simulink model "vectorTest"  (R2020a)
settings: Solver=FixedStepDiscrete  StartTime=0.0  StopTime=10.0  RelTol=1e-3
settings Model: Creator=cyarp  LastModifiedBy=cyarp

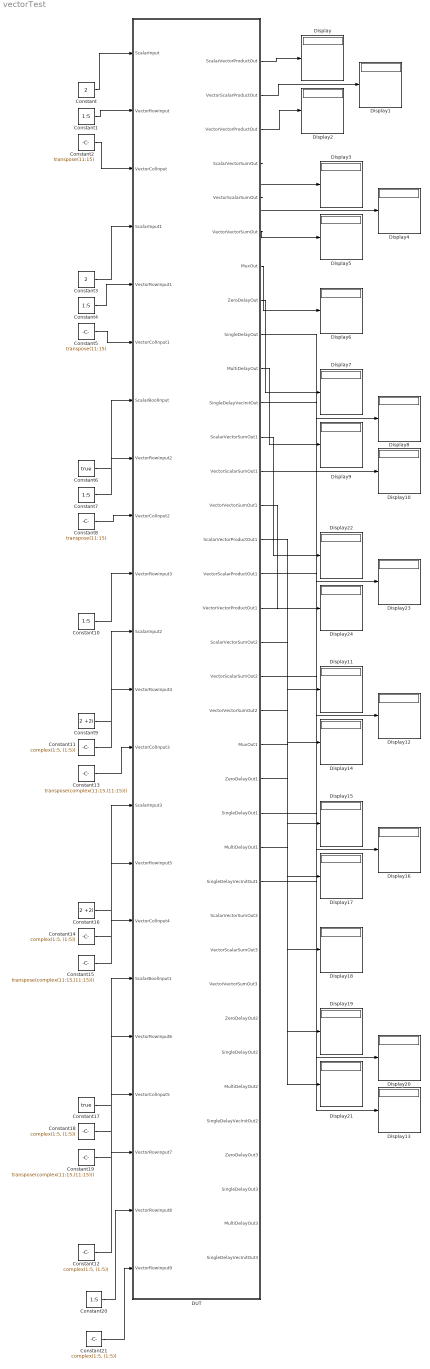
== system vectorTest ==
  Constant : Constant  Value=2
  Constant{1,4,7,10,20} (5 alike) : Constant  Value=1:5
  Constant{11..12,14,18,21} (5 alike) : Constant  Value=complex(1:5, (1:5))
  Constant13 : Constant  Value=transpose(complex(11:15,(11:15)))
  Constant15 : Constant  Value=transpose(complex(11:15,(11:15)))
  Constant16 : Constant  Value=2 +2i
  Constant17 : Constant  Value=true
  Constant19 : Constant  Value=transpose(complex(11:15,(11:15)))
  Constant2 : Constant  Value=transpose(11:15)
  Constant3 : Constant  Value=2
  Constant5 : Constant  Value=transpose(11:15)
  Constant6 : Constant  Value=true
  Constant8 : Constant  Value=transpose(11:15)
  Constant9 : Constant  Value=2 +2i
  DUT : Subsystem
  Display{,1..24} (25 alike) : Display
  wires:
  Constant/1 -> DUT/1(ScalarInput)
  Constant1/1 -> DUT/2(VectorRowInput)
  Constant2/1 -> DUT/3(VectorColInput)
  Constant3/1 -> DUT/4(ScalarInput1)
  Constant4/1 -> DUT/5(VectorRowInput1)
  Constant5/1 -> DUT/6(VectorColInput1)
  Constant6/1 -> DUT/7(ScalarBoolInput)
  Constant7/1 -> DUT/8(VectorRowInput2)
  Constant8/1 -> DUT/9(VectorColInput2)
  Constant10/1 -> DUT/10(VectorRowInput3)
  Constant9/1 -> DUT/11(ScalarInput2)
  Constant11/1 -> DUT/12(VectorRowInput4)
  Constant13/1 -> DUT/13(VectorColInput3)
  Constant16/1 -> DUT/14(ScalarInput3)
  Constant14/1 -> DUT/15(VectorRowInput5)
  Constant15/1 -> DUT/16(VectorColInput4)
  Constant17/1 -> DUT/17(ScalarBoolInput1)
  Constant18/1 -> DUT/18(VectorRowInput6)
  Constant19/1 -> DUT/19(VectorColInput5)
  Constant12/1 -> DUT/20(VectorRowInput7)
  DUT/1(ScalarVectorProductOut) -> Display/1
  DUT/2(VectorScalarProductOut) -> Display1/1
  DUT/3(VectorVectorProductOut) -> Display2/1
  DUT/4(ScalarVectorSumOut) -> Display3/1
  DUT/5(VectorScalarSumOut) -> Display4/1
  DUT/6(VectorVectorSumOut) -> Display5/1
  DUT/7(MuxOut) -> Display6/1
  DUT/8(ZeroDelayOut) -> Display7/1
  DUT/9(SingleDelayOut) -> Display8/1
  DUT/10(MultiDelayOut) -> Display9/1
  DUT/11(SingleDelayVecInitOut) -> Display10/1
  DUT/12(ScalarVectorSumOut1) -> Display22/1
  DUT/13(VectorScalarSumOut1) -> Display23/1
  DUT/14(VectorVectorSumOut1) -> Display24/1
  DUT/15(ScalarVectorProductOut1) -> Display11/1
  DUT/16(VectorScalarProductOut1) -> Display12/1
  DUT/17(VectorVectorProductOut1) -> Display14/1
  DUT/18(ScalarVectorSumOut2) -> Display15/1
  DUT/19(VectorScalarSumOut2) -> Display16/1
  DUT/20(VectorVectorSumOut2) -> Display17/1
  DUT/21(MuxOut1) -> Display18/1
  DUT/22(ZeroDelayOut1) -> Display19/1
  DUT/23(SingleDelayOut1) -> Display20/1
  DUT/24(MultiDelayOut1) -> Display21/1
  DUT/25(SingleDelayVecInitOut1) -> Display13/1
  Constant20/1 -> DUT/21(VectorRowInput8)
  Constant21/1 -> DUT/22(VectorRowInput9)

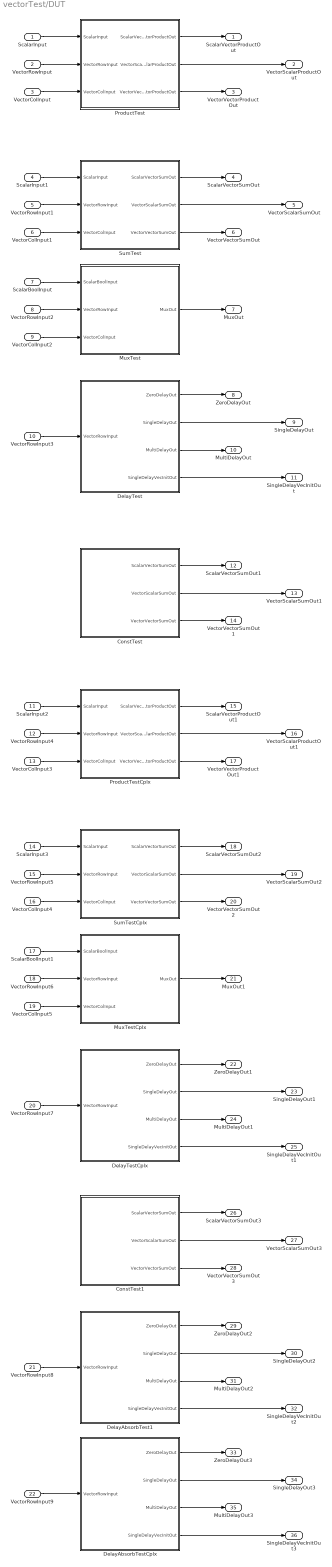
== system vectorTest/DUT ==
  ScalarInput : Inport
  VectorRowInput : Inport  Port=2
  VectorColInput : Inport  Port=3
  ScalarInput1 : Inport  Port=4
  VectorRowInput1 : Inport  Port=5
  VectorColInput1 : Inport  Port=6
  ScalarBoolInput : Inport  Port=7
  VectorRowInput2 : Inport  Port=8
  VectorColInput2 : Inport  Port=9
  VectorRowInput3 : Inport  Port=10
  ScalarInput2 : Inport  Port=11
  VectorRowInput4 : Inport  Port=12
  VectorColInput3 : Inport  Port=13
  ScalarInput3 : Inport  Port=14
  VectorRowInput5 : Inport  Port=15
  VectorColInput4 : Inport  Port=16
  ScalarBoolInput1 : Inport  Port=17
  VectorRowInput6 : Inport  Port=18
  VectorColInput5 : Inport  Port=19
  VectorRowInput7 : Inport  Port=20
  VectorRowInput8 : Inport  Port=21
  VectorRowInput9 : Inport  Port=22
  ConstTest : Subsystem
  ConstTest1 : Subsystem
  DelayAbsorbTest1 : Subsystem
  DelayAbsorbTestCplx : Subsystem
  DelayTest : Subsystem
  DelayTestCplx : Subsystem
  MuxTest : Subsystem
  MuxTestCplx : Subsystem
  ProductTest : Subsystem
  ProductTestCplx : Subsystem
  SumTest : Subsystem
  SumTestCplx : Subsystem
  ScalarVectorProductOut : Outport
  VectorScalarProductOut : Outport  Port=2
  VectorVectorProductOut : Outport  Port=3
  ScalarVectorSumOut : Outport  Port=4
  VectorScalarSumOut : Outport  Port=5
  VectorVectorSumOut : Outport  Port=6
  MuxOut : Outport  Port=7
  ZeroDelayOut : Outport  Port=8
  SingleDelayOut : Outport  Port=9
  MultiDelayOut : Outport  Port=10
  SingleDelayVecInitOut : Outport  Port=11
  ScalarVectorSumOut1 : Outport  Port=12
  VectorScalarSumOut1 : Outport  Port=13
  VectorVectorSumOut1 : Outport  Port=14
  ScalarVectorProductOut1 : Outport  Port=15
  VectorScalarProductOut1 : Outport  Port=16
  VectorVectorProductOut1 : Outport  Port=17
  ScalarVectorSumOut2 : Outport  Port=18
  VectorScalarSumOut2 : Outport  Port=19
  VectorVectorSumOut2 : Outport  Port=20
  MuxOut1 : Outport  Port=21
  ZeroDelayOut1 : Outport  Port=22
  SingleDelayOut1 : Outport  Port=23
  MultiDelayOut1 : Outport  Port=24
  SingleDelayVecInitOut1 : Outport  Port=25
  ScalarVectorSumOut3 : Outport  Port=26
  VectorScalarSumOut3 : Outport  Port=27
  VectorVectorSumOut3 : Outport  Port=28
  ZeroDelayOut2 : Outport  Port=29
  SingleDelayOut2 : Outport  Port=30
  MultiDelayOut2 : Outport  Port=31
  SingleDelayVecInitOut2 : Outport  Port=32
  ZeroDelayOut3 : Outport  Port=33
  SingleDelayOut3 : Outport  Port=34
  MultiDelayOut3 : Outport  Port=35
  SingleDelayVecInitOut3 : Outport  Port=36
  wires:
  ConstTest/2(VectorScalarSumOut) -> VectorScalarSumOut1/1
  ScalarInput2/1 -> ProductTestCplx/1(ScalarInput)
  VectorColInput3/1 -> ProductTestCplx/3(VectorColInput)
  ProductTestCplx/3(VectorVectorProductOut) -> VectorVectorProductOut1/1
  DelayTest/4(SingleDelayVecInitOut) -> SingleDelayVecInitOut/1
  VectorRowInput/1 -> ProductTest/2(VectorRowInput)
  ProductTest/3(VectorVectorProductOut) -> VectorVectorProductOut/1
  ProductTest/2(VectorScalarProductOut) -> VectorScalarProductOut/1
  DelayTestCplx/3(MultiDelayOut) -> MultiDelayOut1/1
  ScalarInput1/1 -> SumTest/1(ScalarInput)
  VectorColInput5/1 -> MuxTestCplx/3(VectorColInput)
  VectorColInput2/1 -> MuxTest/3(VectorColInput)
  SumTestCplx/1(ScalarVectorSumOut) -> ScalarVectorSumOut2/1
  SumTestCplx/3(VectorVectorSumOut) -> VectorVectorSumOut2/1
  ProductTest/1(ScalarVectorProductOut) -> ScalarVectorProductOut/1
  VectorColInput4/1 -> SumTestCplx/3(VectorColInput)
  DelayTestCplx/1(ZeroDelayOut) -> ZeroDelayOut1/1
  ConstTest/1(ScalarVectorSumOut) -> ScalarVectorSumOut1/1
  SumTest/1(ScalarVectorSumOut) -> ScalarVectorSumOut/1
  ScalarInput/1 -> ProductTest/1(ScalarInput)
  VectorRowInput1/1 -> SumTest/2(VectorRowInput)
  VectorRowInput3/1 -> DelayTest/1(VectorRowInput)
  DelayTestCplx/4(SingleDelayVecInitOut) -> SingleDelayVecInitOut1/1
  DelayTest/2(SingleDelayOut) -> SingleDelayOut/1
  DelayTest/1(ZeroDelayOut) -> ZeroDelayOut/1
  ConstTest/3(VectorVectorSumOut) -> VectorVectorSumOut1/1
  MuxTest/1(MuxOut) -> MuxOut/1
  VectorRowInput4/1 -> ProductTestCplx/2(VectorRowInput)
  VectorRowInput6/1 -> MuxTestCplx/2(VectorRowInput)
  VectorColInput1/1 -> SumTest/3(VectorColInput)
  ScalarBoolInput/1 -> MuxTest/1(ScalarBoolInput)
  VectorRowInput2/1 -> MuxTest/2(VectorRowInput)
  MuxTestCplx/1(MuxOut) -> MuxOut1/1
  SumTest/3(VectorVectorSumOut) -> VectorVectorSumOut/1
  VectorRowInput5/1 -> SumTestCplx/2(VectorRowInput)
  ScalarInput3/1 -> SumTestCplx/1(ScalarInput)
  SumTest/2(VectorScalarSumOut) -> VectorScalarSumOut/1
  DelayTest/3(MultiDelayOut) -> MultiDelayOut/1
  ProductTestCplx/1(ScalarVectorProductOut) -> ScalarVectorProductOut1/1
  VectorColInput/1 -> ProductTest/3(VectorColInput)
  SumTestCplx/2(VectorScalarSumOut) -> VectorScalarSumOut2/1
  ScalarBoolInput1/1 -> MuxTestCplx/1(ScalarBoolInput)
  ProductTestCplx/2(VectorScalarProductOut) -> VectorScalarProductOut1/1
  VectorRowInput7/1 -> DelayTestCplx/1(VectorRowInput)
  DelayTestCplx/2(SingleDelayOut) -> SingleDelayOut1/1
  ConstTest1/1(ScalarVectorSumOut) -> ScalarVectorSumOut3/1
  ConstTest1/2(VectorScalarSumOut) -> VectorScalarSumOut3/1
  ConstTest1/3(VectorVectorSumOut) -> VectorVectorSumOut3/1
  VectorRowInput8/1 -> DelayAbsorbTest1/1(VectorRowInput)
  DelayAbsorbTest1/2(SingleDelayOut) -> SingleDelayOut2/1
  DelayAbsorbTest1/1(ZeroDelayOut) -> ZeroDelayOut2/1
  DelayAbsorbTest1/3(MultiDelayOut) -> MultiDelayOut2/1
  DelayAbsorbTest1/4(SingleDelayVecInitOut) -> SingleDelayVecInitOut2/1
  DelayAbsorbTestCplx/1(ZeroDelayOut) -> ZeroDelayOut3/1
  DelayAbsorbTestCplx/2(SingleDelayOut) -> SingleDelayOut3/1
  VectorRowInput9/1 -> DelayAbsorbTestCplx/1(VectorRowInput)
  DelayAbsorbTestCplx/4(SingleDelayVecInitOut) -> SingleDelayVecInitOut3/1
  DelayAbsorbTestCplx/3(MultiDelayOut) -> MultiDelayOut3/1

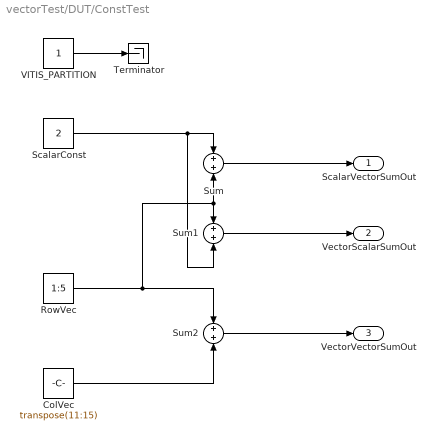
== system vectorTest/DUT/ConstTest ==
  ColVec : Constant  Value=transpose(11:15)
  RowVec : Constant  Value=1:5
  ScalarConst : Constant  Value=2
  Sum : Sum
  Sum1 : Sum
  Sum2 : Sum
  Terminator : Terminator
  VITIS_PARTITION : Constant
  ScalarVectorSumOut : Outport
  VectorScalarSumOut : Outport  Port=2
  VectorVectorSumOut : Outport  Port=3
  wires:
  ScalarConst/1 -> Sum1/2, Sum/1
  RowVec/1 -> Sum2/1, Sum1/1, Sum/2
  ColVec/1 -> Sum2/2
  Sum/1 -> ScalarVectorSumOut/1
  Sum1/1 -> VectorScalarSumOut/1
  Sum2/1 -> VectorVectorSumOut/1
  VITIS_PARTITION/1 -> Terminator/1

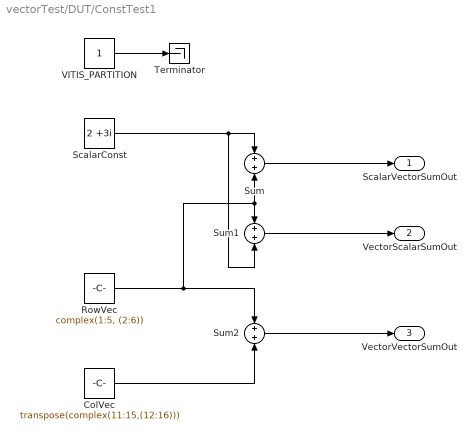
== system vectorTest/DUT/ConstTest1 ==
  ColVec : Constant  Value=transpose(complex(11:15,(12:16)))
  RowVec : Constant  Value=complex(1:5, (2:6))
  ScalarConst : Constant  Value=2 +3i
  Sum : Sum
  Sum1 : Sum
  Sum2 : Sum
  Terminator : Terminator
  VITIS_PARTITION : Constant
  ScalarVectorSumOut : Outport
  VectorScalarSumOut : Outport  Port=2
  VectorVectorSumOut : Outport  Port=3
  wires:
  ScalarConst/1 -> Sum1/2, Sum/1
  RowVec/1 -> Sum2/1, Sum1/1, Sum/2
  ColVec/1 -> Sum2/2
  Sum/1 -> ScalarVectorSumOut/1
  Sum1/1 -> VectorScalarSumOut/1
  Sum2/1 -> VectorVectorSumOut/1
  VITIS_PARTITION/1 -> Terminator/1

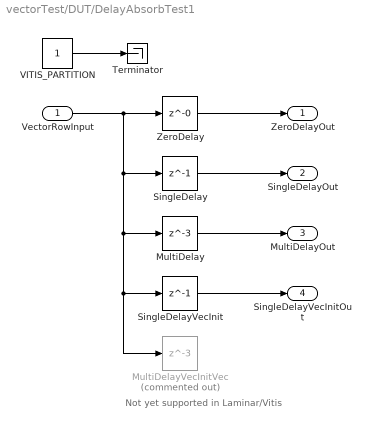
== system vectorTest/DUT/DelayAbsorbTest1 ==
  note: Not yet supported in Laminar/Vitis
  VectorRowInput : Inport
  MultiDelay : Delay  DelayLength=3
  MultiDelayVecInitVec : Delay  Commented=on  DelayLength=3  InitialCondition=transpose([6, 7, 8, 9, 10; 3, 4, 5, 6, 7; 11, 22, 33, 44, 55])
  SingleDelay : Delay  DelayLength=1
  SingleDelayVecInit : Delay  DelayLength=1  InitialCondition=[6, 7, 8, 9, 10]
  Terminator : Terminator
  VITIS_PARTITION : Constant
  ZeroDelay : Delay  DelayLength=0
  ZeroDelayOut : Outport
  SingleDelayOut : Outport  Port=2
  MultiDelayOut : Outport  Port=3
  SingleDelayVecInitOut : Outport  Port=4
  wires:
  ZeroDelay/1 -> ZeroDelayOut/1
  VectorRowInput/1 -> MultiDelayVecInitVec/1, SingleDelayVecInit/1, MultiDelay/1, SingleDelay/1, ZeroDelay/1
  SingleDelay/1 -> SingleDelayOut/1
  MultiDelay/1 -> MultiDelayOut/1
  SingleDelayVecInit/1 -> SingleDelayVecInitOut/1
  VITIS_PARTITION/1 -> Terminator/1

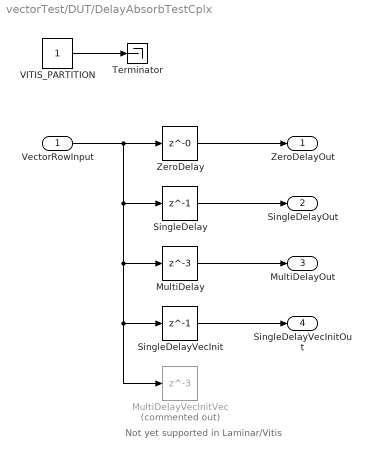
== system vectorTest/DUT/DelayAbsorbTestCplx ==
  note: Not yet supported in Laminar/Vitis
  VectorRowInput : Inport
  MultiDelay : Delay  DelayLength=3
  MultiDelayVecInitVec : Delay  Commented=on  DelayLength=3  InitialCondition=transpose([6, 7, 8, 9, 10; 3, 4, 5, 6, 7; 11, 22, 33, 44, 55])
  SingleDelay : Delay  DelayLength=1
  SingleDelayVecInit : Delay  DelayLength=1  InitialCondition=[6, 7, 8, 9, 10]
  Terminator : Terminator
  VITIS_PARTITION : Constant
  ZeroDelay : Delay  DelayLength=0
  ZeroDelayOut : Outport
  SingleDelayOut : Outport  Port=2
  MultiDelayOut : Outport  Port=3
  SingleDelayVecInitOut : Outport  Port=4
  wires:
  ZeroDelay/1 -> ZeroDelayOut/1
  VectorRowInput/1 -> MultiDelayVecInitVec/1, SingleDelayVecInit/1, MultiDelay/1, SingleDelay/1, ZeroDelay/1
  SingleDelay/1 -> SingleDelayOut/1
  MultiDelay/1 -> MultiDelayOut/1
  SingleDelayVecInit/1 -> SingleDelayVecInitOut/1
  VITIS_PARTITION/1 -> Terminator/1

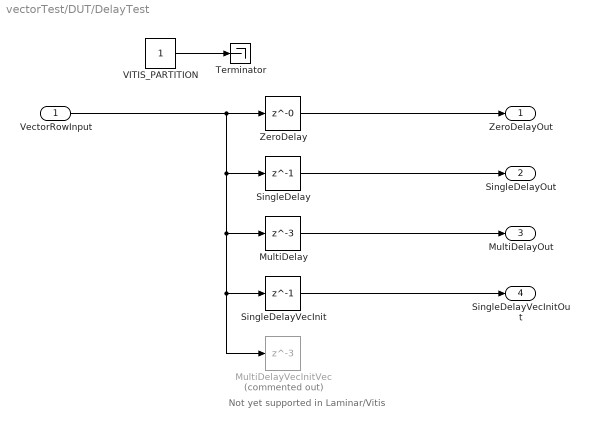
== system vectorTest/DUT/DelayTest ==
  note: Not yet supported in Laminar/Vitis
  VectorRowInput : Inport
  MultiDelay : Delay  DelayLength=3
  MultiDelayVecInitVec : Delay  Commented=on  DelayLength=3  InitialCondition=transpose([6, 7, 8, 9, 10; 3, 4, 5, 6, 7; 11, 22, 33, 44, 55])
  SingleDelay : Delay  DelayLength=1
  SingleDelayVecInit : Delay  DelayLength=1  InitialCondition=[6, 7, 8, 9, 10]
  Terminator : Terminator
  VITIS_PARTITION : Constant
  ZeroDelay : Delay  DelayLength=0
  ZeroDelayOut : Outport
  SingleDelayOut : Outport  Port=2
  MultiDelayOut : Outport  Port=3
  SingleDelayVecInitOut : Outport  Port=4
  wires:
  VITIS_PARTITION/1 -> Terminator/1
  VectorRowInput/1 -> MultiDelayVecInitVec/1, SingleDelayVecInit/1, MultiDelay/1, SingleDelay/1, ZeroDelay/1
  ZeroDelay/1 -> ZeroDelayOut/1
  SingleDelay/1 -> SingleDelayOut/1
  MultiDelay/1 -> MultiDelayOut/1
  SingleDelayVecInit/1 -> SingleDelayVecInitOut/1

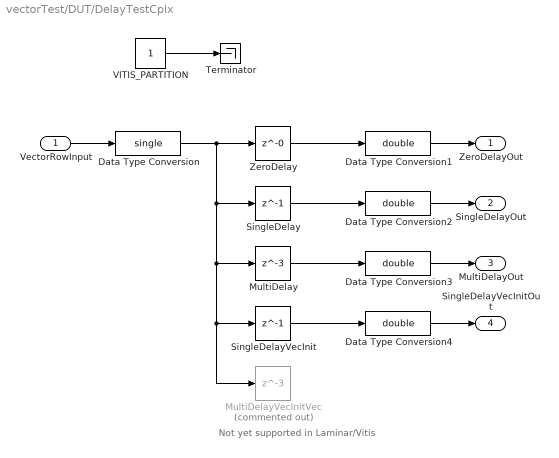
== system vectorTest/DUT/DelayTestCplx ==
  note: Not yet supported in Laminar/Vitis
  VectorRowInput : Inport
  Data Type Conversion : DataTypeConversion  OutDataTypeStr=single
  Data Type Conversion{1..4} (4 alike) : DataTypeConversion  OutDataTypeStr=double
  MultiDelay : Delay  DelayLength=3
  MultiDelayVecInitVec : Delay  Commented=on  DelayLength=3  InitialCondition=transpose([6, 7, 8, 9, 10; 3, 4, 5, 6, 7; 11, 22, 33, 44, 55])
  SingleDelay : Delay  DelayLength=1
  SingleDelayVecInit : Delay  DelayLength=1  InitialCondition=[6, 7, 8, 9, 10]
  Terminator : Terminator
  VITIS_PARTITION : Constant
  ZeroDelay : Delay  DelayLength=0
  ZeroDelayOut : Outport
  SingleDelayOut : Outport  Port=2
  MultiDelayOut : Outport  Port=3
  SingleDelayVecInitOut : Outport  Port=4
  wires:
  ZeroDelay/1 -> Data Type Conversion1/1
  VectorRowInput/1 -> Data Type Conversion/1
  SingleDelay/1 -> Data Type Conversion2/1
  MultiDelay/1 -> Data Type Conversion3/1
  SingleDelayVecInit/1 -> Data Type Conversion4/1
  VITIS_PARTITION/1 -> Terminator/1
  Data Type Conversion/1 -> MultiDelayVecInitVec/1, SingleDelayVecInit/1, MultiDelay/1, SingleDelay/1, ZeroDelay/1
  Data Type Conversion1/1 -> ZeroDelayOut/1
  Data Type Conversion2/1 -> SingleDelayOut/1
  Data Type Conversion3/1 -> MultiDelayOut/1
  Data Type Conversion4/1 -> SingleDelayVecInitOut/1

== system vectorTest/DUT/MuxTest ==
  ScalarBoolInput : Inport  OutDataTypeStr=boolean
  VectorRowInput : Inport  Port=2
  VectorColInput : Inport  Port=3
  Switch : Switch  Criteria=u2 ~= 0
  Terminator : Terminator
  VITIS_PARTITION : Constant
  MuxOut : Outport
  wires:
  VectorRowInput/1 -> Switch/1
  VectorColInput/1 -> Switch/3
  ScalarBoolInput/1 -> Switch/2
  Switch/1 -> MuxOut/1
  VITIS_PARTITION/1 -> Terminator/1

== system vectorTest/DUT/MuxTestCplx ==
  ScalarBoolInput : Inport  OutDataTypeStr=boolean
  VectorRowInput : Inport  Port=2
  VectorColInput : Inport  Port=3
  Switch : Switch  Criteria=u2 ~= 0
  Terminator : Terminator
  VITIS_PARTITION : Constant
  MuxOut : Outport
  wires:
  VectorRowInput/1 -> Switch/1
  VectorColInput/1 -> Switch/3
  ScalarBoolInput/1 -> Switch/2
  Switch/1 -> MuxOut/1
  VITIS_PARTITION/1 -> Terminator/1

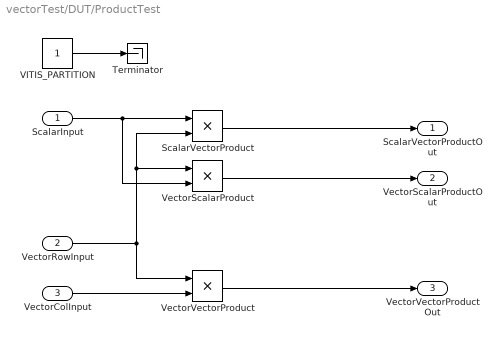
== system vectorTest/DUT/ProductTest ==
  ScalarInput : Inport
  VectorRowInput : Inport  Port=2
  VectorColInput : Inport  Port=3
  ScalarVectorProduct : Product
  Terminator : Terminator
  VITIS_PARTITION : Constant
  VectorScalarProduct : Product
  VectorVectorProduct : Product
  ScalarVectorProductOut : Outport
  VectorScalarProductOut : Outport  Port=2
  VectorVectorProductOut : Outport  Port=3
  wires:
  ScalarInput/1 -> VectorScalarProduct/2, ScalarVectorProduct/1
  VectorRowInput/1 -> VectorScalarProduct/1, ScalarVectorProduct/2, VectorVectorProduct/1
  VectorColInput/1 -> VectorVectorProduct/2
  ScalarVectorProduct/1 -> ScalarVectorProductOut/1
  VectorScalarProduct/1 -> VectorScalarProductOut/1
  VectorVectorProduct/1 -> VectorVectorProductOut/1
  VITIS_PARTITION/1 -> Terminator/1

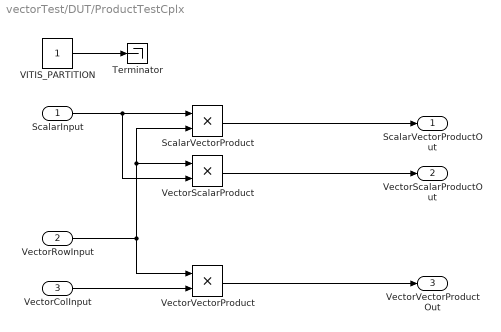
== system vectorTest/DUT/ProductTestCplx ==
  ScalarInput : Inport
  VectorRowInput : Inport  Port=2
  VectorColInput : Inport  Port=3
  ScalarVectorProduct : Product
  Terminator : Terminator
  VITIS_PARTITION : Constant
  VectorScalarProduct : Product
  VectorVectorProduct : Product
  ScalarVectorProductOut : Outport
  VectorScalarProductOut : Outport  Port=2
  VectorVectorProductOut : Outport  Port=3
  wires:
  ScalarInput/1 -> VectorScalarProduct/2, ScalarVectorProduct/1
  VectorRowInput/1 -> VectorScalarProduct/1, ScalarVectorProduct/2, VectorVectorProduct/1
  VectorColInput/1 -> VectorVectorProduct/2
  ScalarVectorProduct/1 -> ScalarVectorProductOut/1
  VectorScalarProduct/1 -> VectorScalarProductOut/1
  VectorVectorProduct/1 -> VectorVectorProductOut/1
  VITIS_PARTITION/1 -> Terminator/1

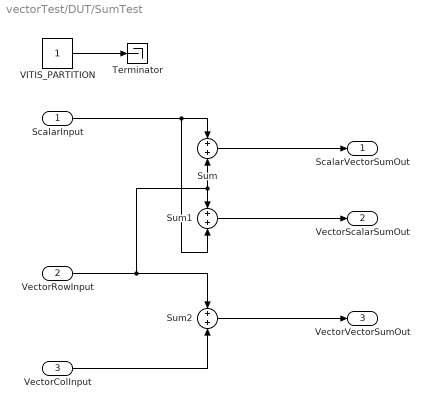
== system vectorTest/DUT/SumTest ==
  ScalarInput : Inport
  VectorRowInput : Inport  Port=2
  VectorColInput : Inport  Port=3
  Sum : Sum
  Sum1 : Sum
  Sum2 : Sum
  Terminator : Terminator
  VITIS_PARTITION : Constant
  ScalarVectorSumOut : Outport
  VectorScalarSumOut : Outport  Port=2
  VectorVectorSumOut : Outport  Port=3
  wires:
  ScalarInput/1 -> Sum1/2, Sum/1
  VectorRowInput/1 -> Sum2/1, Sum1/1, Sum/2
  VectorColInput/1 -> Sum2/2
  Sum/1 -> ScalarVectorSumOut/1
  Sum1/1 -> VectorScalarSumOut/1
  Sum2/1 -> VectorVectorSumOut/1
  VITIS_PARTITION/1 -> Terminator/1

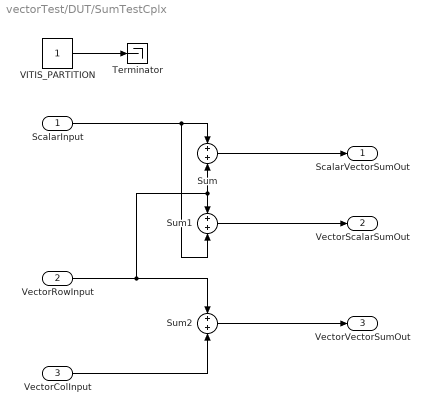
== system vectorTest/DUT/SumTestCplx ==
  ScalarInput : Inport
  VectorRowInput : Inport  Port=2
  VectorColInput : Inport  Port=3
  Sum : Sum
  Sum1 : Sum
  Sum2 : Sum
  Terminator : Terminator
  VITIS_PARTITION : Constant
  ScalarVectorSumOut : Outport
  VectorScalarSumOut : Outport  Port=2
  VectorVectorSumOut : Outport  Port=3
  wires:
  ScalarInput/1 -> Sum1/2, Sum/1
  VectorRowInput/1 -> Sum2/1, Sum1/1, Sum/2
  VectorColInput/1 -> Sum2/2
  Sum/1 -> ScalarVectorSumOut/1
  Sum1/1 -> VectorScalarSumOut/1
  Sum2/1 -> VectorVectorSumOut/1
  VITIS_PARTITION/1 -> Terminator/1
